simulink model "untitled"  (R2020a)
settings: Solver=FixedStepAuto  StartTime=0.0  StopTime=100000  FixedStep=1/100  RelTol=1e-3
libraries: robotmobilelib x1
settings Model: Creator=Peter  LastModifiedBy=Peter

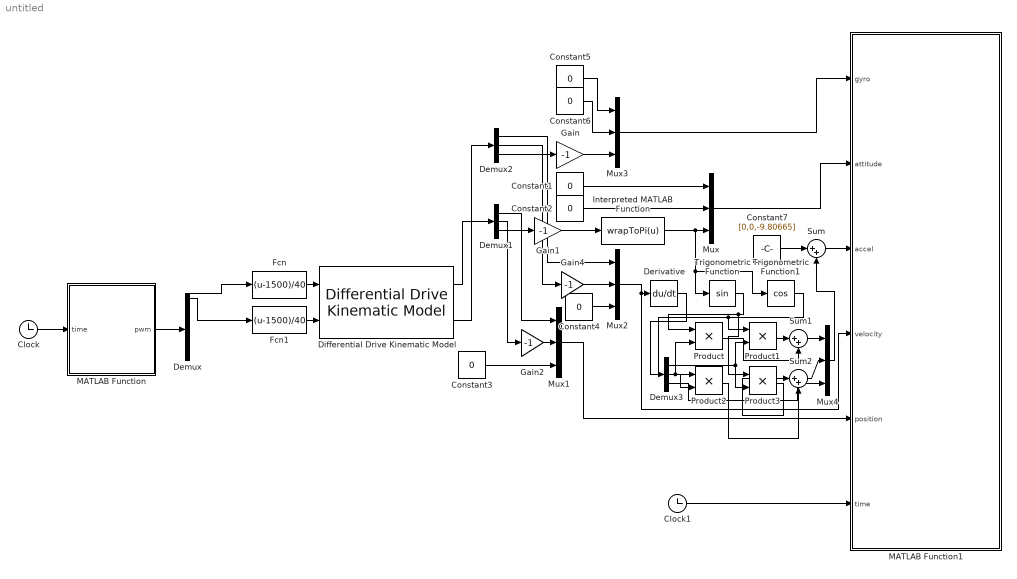
== system untitled ==
  Clock : Clock
  Clock1 : Clock
  Constant{1..6} (6 alike) : Constant  Value=0
  Constant7 : Constant  Value=[0,0,-9.80665]
  Demux : Demux  Outputs=16
  Demux1 : Demux  Outputs=3
  Demux2 : Demux  Outputs=3
  Demux3 : Demux  Outputs=3
  Derivative : Derivative
  Differential Drive Kinematic Model : robotmobilelib/Differential Drive Kinematic Model  VehicleInputs=Wheel Speeds  WheelRadius=0.16  WheelSpeedRange=[-100 100]  TrackWidth=0.2  InitialState=[0; 0; 0]  SimulateUsing=Interpreted execution
      settings: SourceProductBaseCode=RO
  Fcn : Fcn  Expr=(u-1500)/40
  Fcn1 : Fcn  Expr=(u-1500)/40
  Gain{,1..2,4} (4 alike) : Gain  Gain=-1
  Interpreted MATLAB Function : MATLABFcn  MATLABFcn=wrapToPi(u)
  MATLAB Function : MATLAB Function  TreatAsAtomicUnit=on
  MATLAB Function1 : MATLAB Function  TreatAsAtomicUnit=on
  Mux{,1..4} (5 alike) : Mux  Inputs=3
  Product{,1..3} (4 alike) : Product
  Sum : Sum  Inputs=|++
  Sum1 : Sum  Inputs=|++
  Sum2 : Sum  Inputs=|++
  Trigonometric Function : Trigonometry
  Trigonometric Function1 : Trigonometry  Operator=cos
  wires:
  Demux/2 -> Fcn1/1
  MATLAB Function/1(pwm) -> Demux/1
  Fcn/1 -> Differential Drive Kinematic Model/1
  Clock/1 -> MATLAB Function/1(time)
  Demux/1 -> Fcn/1
  Fcn1/1 -> Differential Drive Kinematic Model/2
  Clock1/1 -> MATLAB Function1/6(time)
  Differential Drive Kinematic Model/1 -> Demux1/1
  Demux1/3 -> Gain1/1
  Mux/1 -> MATLAB Function1/2(attitude)
  Constant1/1 -> Mux/1
  Constant2/1 -> Mux/2
  Mux1/1 -> MATLAB Function1/5(position)
  Demux1/2 -> Gain2/1
  Constant3/1 -> Mux1/3
  Differential Drive Kinematic Model/2 -> Demux2/1
  Constant4/1 -> Mux2/3
  Demux2/2 -> Gain4/1
  Demux2/1 -> Mux2/1
  Mux3/1 -> MATLAB Function1/1(gyro)
  Constant6/1 -> Mux3/2
  Constant5/1 -> Mux3/1
  Demux2/3 -> Gain/1
  Mux2/1 -> Derivative/1, MATLAB Function1/4(velocity)
  Constant7/1 -> Sum/1
  Gain/1 -> Mux3/3
  Gain1/1 -> Interpreted MATLAB Function/1
  Demux1/1 -> Mux1/1
  Gain2/1 -> Mux1/2
  Interpreted MATLAB Function/1 -> Trigonometric Function/1, Trigonometric Function1/1, Mux/3
  Gain4/1 -> Mux2/2
  Sum/1 -> MATLAB Function1/3(accel)
  Derivative/1 -> Demux3/1
  Demux3/2 -> Product/2, Product2/2
  Trigonometric Function/1 -> Product3/1, Product/1
  Demux3/1 -> Product1/2, Product3/2
  Mux4/1 -> Sum/2
  Demux3/3 -> Mux4/3
  Trigonometric Function1/1 -> Product1/1, Product2/1
  Product1/1 -> Sum1/1
  Sum1/1 -> Mux4/1
  Product/1 -> Sum1/2
  Product3/1 -> Sum2/1
  Sum2/1 -> Mux4/2
  Product2/1 -> Sum2/2

== matlab function untitled/MATLAB Function1 ==
  data: gyro input; attitude input; accel input; velocity input; position input; time input
function fcn(gyro, attitude, accel, velocity, position, time)
coder.extrinsic('AP_send')
AP_send(gyro, attitude, accel, velocity, position, time)
end

== matlab function untitled/MATLAB Function ==
  data: pwm output; time input
function pwm  = fcn(time)
pwm = zeros(16,1);
coder.extrinsic('AP_receve')
pwm = AP_receve(time);
end
